simulink subsystem "to_complex"  (R2021b)
settings: Solver=VariableStepAuto  StartTime=0.0  StopTime=10.0  RelTol=1e-3
settings Model: Creator=torha  LastModifiedBy=torha

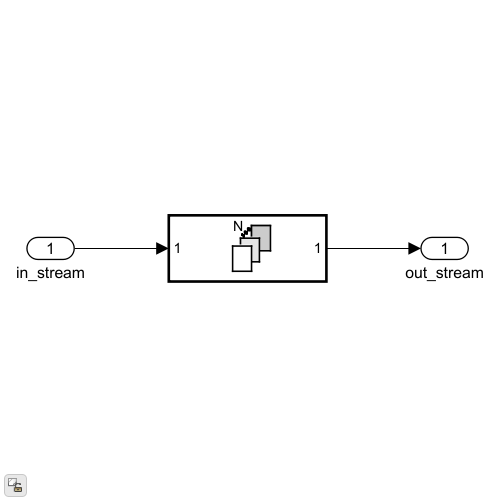
[thumbnail: Simulink's stored preview of the top-level diagram]
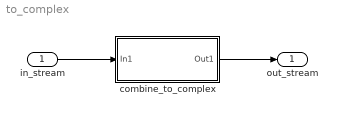
== system to_complex ==
  in_stream : Inport
  combine_to_complex : Subsystem  TreatAsAtomicUnit=on
  out_stream : Outport
  wires:
  combine_to_complex/1(Out1) -> out_stream/1
  in_stream/1 -> combine_to_complex/1(In1)

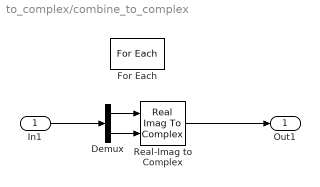
== system to_complex/combine_to_complex ==
  In1 : Inport  Partition=on  PartitionDimension=2  PartitionWidth=2  PartitionOffset=0
  Demux : Demux  Outputs=2
  For Each : ForEach  DisableCoverage=on
  Real-Imag to Complex : RealImagToComplex
  Out1 : Outport  ConcatenationDimension=2
  wires:
  Demux/1 -> Real-Imag to Complex/1
  Demux/2 -> Real-Imag to Complex/2
  Real-Imag to Complex/1 -> Out1/1
  In1/1 -> Demux/1
